simulink model "invertedpend"  (R2021a)
settings: Solver=FixedStepAuto  StartTime=0.0  StopTime=5  FixedStep=0.01  RelTol=1e-3
values from neighbouring files (symbols this model uses):
  bc = 0.1    [invertedPenMotor.m]    (also in invertedStateSpace.m)
  bp = 0.005    [invertedPenMotor.m]    (also in invertedStateSpace.m = 0)
  g = 9.81    [invertedPenMotor.m]    (also in invertedStateSpace.m)
  I = 0.01    [invertedPenMotor.m]    (also in invertedStateSpace.m)
  k = lqr(A,B,Q,R)    [invertedPenMotor.m]    (also in invertedStateSpace.m)
  l = 0.6    [invertedPenMotor.m]    (also in invertedStateSpace.m)
  mc = 0.75    [invertedPenMotor.m]    (also in invertedStateSpace.m)
  mp = 0.5    [invertedPenMotor.m]    (also in invertedStateSpace.m)
  Nbar = Nu + k*Nx    [invertedPenMotor.m]    (also in invertedStateSpace.m)
settings Model: Creator=hussein  LastModifiedBy=hussein

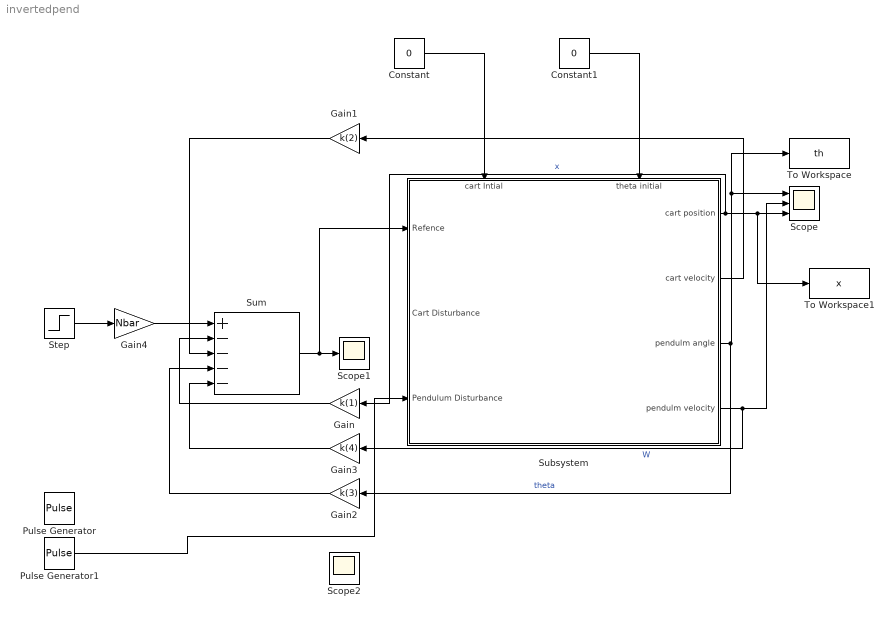
== system invertedpend ==
  Constant : Constant  Value=0
  Constant1 : Constant  Value=0
  Gain : Gain  Gain=k(1)
  Gain1 : Gain  Gain=k(2)
  Gain2 : Gain  Gain=k(3)
  Gain3 : Gain  Gain=k(4)
  Gain4 : Gain  Gain=Nbar
  Pulse Generator : DiscretePulseGenerator  PulseType=Time based  Amplitude=25  Period=5  PhaseDelay=2.5
  Pulse Generator1 : DiscretePulseGenerator  PulseType=Time based  Amplitude=25  Period=5  PhaseDelay=2.5
  Scope : Scope  NumInputPorts=3
  Scope1 : Scope
  Scope2 : Scope
  Step : Step  Time=0  After=0.25  SampleTime=0
  Subsystem : Subsystem
      settings: PortSchema="{\"entries\":[{\"content\":{\"sides\":[{\"content\":{\"connectorIds\":[\"In1\",\"In2\",\"In3\"]},\"type\":\"ConnectorPlacement.EquallySpacedRectSide\",\"uuid\":\"a94d039f-07dc-4bfd-b7f7-29099b730fb6\"},{\"content\":{\"connectorIds\":[\"Out1\",\"Out2\",\"Out3\",\"Out4\"],\"side\":\"RIGHT\"},\"type\":\"ConnectorPlacement.EquallySpacedRectSide\",\"uuid\":\"57859fac-5407-4f7b-91db-7d1251c57063\"},{\"content\":{\"connectorIds\":[\"In4\",\"In5\"],\"side\":\"TOP\"},\"type\":\"ConnectorPlacement.EquallySpacedRectSide\",\"uuid\":\"3a84473e-639c-43f1-96b8-92ab0687d4a5\"},{\"content\":{\"connectorIds\":[],\"side\":\"BOTTOM\"},\"type\":\"ConnectorPlacement.EquallySpacedRectSide\",\"uuid\":\"bdd9be4c-c5e0-46e4-aa97-fa103129b5ab\"}]},\"type\":\"ConnectorPlacement.EquallySpacedConnector\",\"uuid\":\"77cd2099-948c-49fd-a523-d060646d1b88\"}],\"packageUris\":[\"http://schema.mathworks.com/mf0/Connector/R2020b\"],\"version\":\"1.0\"}"
  Sum : Sum  Inputs=+----
  To Workspace : ToWorkspace  VariableName=th  SaveFormat=Timeseries  SampleTime=-1
  To Workspace1 : ToWorkspace  VariableName=x  SaveFormat=Timeseries  SampleTime=-1
  wires:
  Subsystem/2(cart velocity) -> Gain1/1
  Gain/1 -> Sum/2
  Gain1/1 -> Sum/3
  Gain2/1 -> Sum/4
  Subsystem/4(pendulm velocity) -> Scope/2, Gain3/1  "W"
  Gain3/1 -> Sum/5
  Subsystem/1(cart position) -> To Workspace1/1, Scope/3, Gain/1  "x"
  Gain4/1 -> Sum/1
  Subsystem/3(pendulm angle) -> Scope/1, To Workspace/1, Gain2/1  "theta"
  Step/1 -> Gain4/1
  Sum/1 -> Scope1/1, Subsystem/1(Refence)
  Constant/1 -> Subsystem/4(cart Intial)
  Constant1/1 -> Subsystem/5(theta initial)
  Pulse Generator1/1 -> Subsystem/3(Pendulum Disturbance)

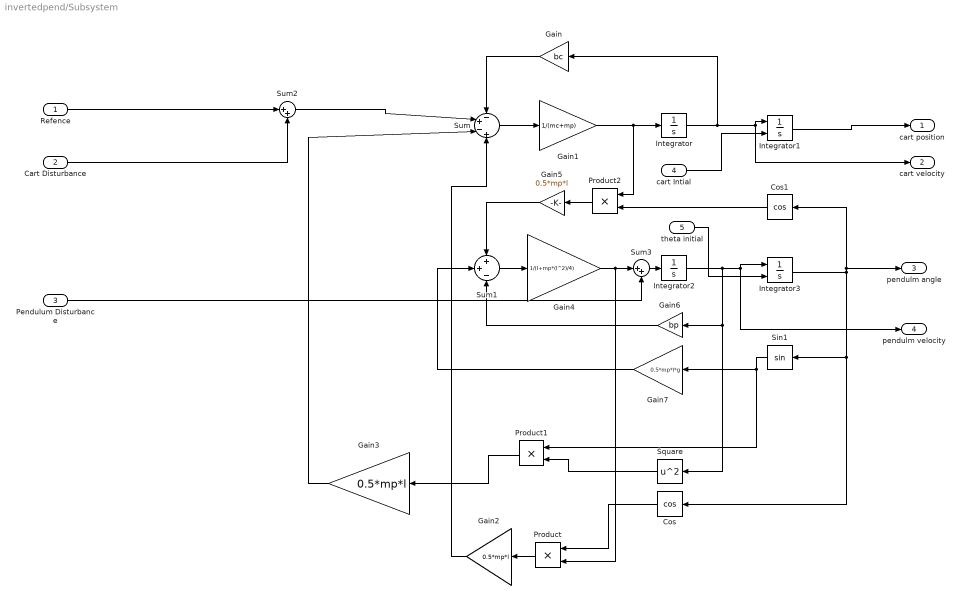
== system invertedpend/Subsystem ==
  Refence : Inport
  Cart Disturbance : Inport  Port=2
  Pendulum Disturbance : Inport  Port=3
  cart Intial : Inport  Port=4
  theta initial : Inport  Port=5
  Cos : Trigonometry  Operator=cos
  Cos1 : Trigonometry  Operator=cos
  Gain : Gain  Gain=bc
  Gain1 : Gain  Gain=1/(mc+mp)
  Gain2 : Gain  Gain=0.5*mp*l
  Gain3 : Gain  Gain=0.5*mp*l
  Gain4 : Gain  Gain=1/(I+mp*(l^2)/4)
  Gain5 : Gain  Gain=0.5*mp*l
  Gain6 : Gain  Gain=bp
  Gain7 : Gain  Gain=0.5*mp*l*g
  Integrator : Integrator
  Integrator1 : Integrator  InitialConditionSource=external
  Integrator2 : Integrator
  Integrator3 : Integrator  InitialConditionSource=external
  Product : Product
  Product1 : Product
  Product2 : Product
  Sin1 : Trigonometry
  Square : Math  Operator=square  SaturateOnIntegerOverflow=on
  Sum : Sum  Inputs=-+-+
  Sum1 : Sum  Inputs=++-
  Sum2 : Sum  Inputs=|++
  Sum3 : Sum  Inputs=|++
  cart position : Outport
  cart velocity : Outport  Port=2
  pendulm angle : Outport  Port=3
  pendulm velocity : Outport  Port=4
  wires:
  Gain1/1 -> Product2/1, Integrator/1
  Product/1 -> Gain2/1
  Gain6/1 -> Sum1/3
  Integrator2/1 -> Square/1, Gain6/1, pendulm velocity/1, Integrator3/1
  Product1/1 -> Gain3/1
  Gain2/1 -> Sum/4
  Cos/1 -> Product/1
  Cos1/1 -> Product2/2
  Sum/1 -> Gain1/1
  Gain3/1 -> Sum/3
  Sum1/1 -> Gain4/1
  Gain/1 -> Sum/1
  Gain5/1 -> Sum1/1
  Product2/1 -> Gain5/1
  Gain7/1 -> Sum1/2
  Integrator1/1 -> cart position/1
  Integrator/1 -> Gain/1, cart velocity/1, Integrator1/1
  Sin1/1 -> Product1/1, Gain7/1
  Square/1 -> Product1/2
  Refence/1 -> Sum2/1
  Cart Disturbance/1 -> Sum2/2
  Sum2/1 -> Sum/2
  Gain4/1 -> Sum3/1, Product/2
  Integrator3/1 -> Cos1/1, pendulm angle/1, Cos/1, Sin1/1
  Sum3/1 -> Integrator2/1
  Pendulum Disturbance/1 -> Sum3/2
  cart Intial/1 -> Integrator1/2
  theta initial/1 -> Integrator3/2
